simulink model "Damping_model"  (R2020a)
settings: Solver=VariableStepAuto  StartTime=0.0  StopTime=5  RelTol=1e-3  AbsTol=1e-3
undefined symbols (not defined in the file): b, b1, b2, b3, k, m
libraries: fl_lib x6, nesl_utility x3
settings Model: Creator=vltn0  LastModifiedBy=vltn0
settings SolverCC: AutoScaleAbsTol=off
settings DebuggingCC: SymbolicDimsDataTypeCodeGenerationDiagnostic=none
settings SFSimCC: CustomCodeUndefinedFunction=UseInterfaceOnly
settings SimscapeCC: SimscapeLogType=all  SimscapeLogSimulationStatistics=on  SimscapeLogDataHistory=10000

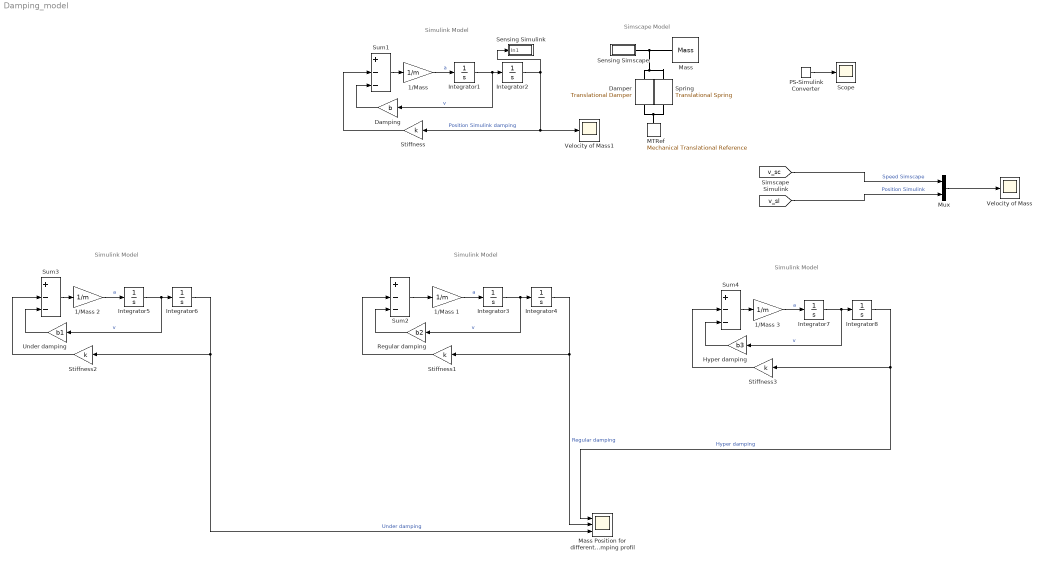
== system Damping_model ==
  note: Simulink Model
  note: Simscape Model
  note: Simulink Model
  note: Simulink Model
  note: Simulink Model
  1/Mass {,1..3} (4 alike) : Gain  Gain=1/m  SaturateOnIntegerOverflow=on  OutDataTypeStr=Inherit: Same as input  ParamDataTypeStr=Inherit: Same as input
  Damper : fl_lib/Mechanical/Translational Elements/Translational Damper  D=b N/(m/s)  v_specify=off  v_priority=High  v=0 m/s  v_nominal_specify=off  v_nominal_unit=m/s  v_nominal_value=1  f_specify=off  f_priority=High  f=0 N  f_nominal_specify=off  f_nominal_unit=N  f_nominal_value=1
  Damping : Gain  Gain=b  SaturateOnIntegerOverflow=on  OutDataTypeStr=Inherit: Same as input  ParamDataTypeStr=Inherit: Same as input
  Hyper damping : Gain  Gain=b3  SaturateOnIntegerOverflow=on  OutDataTypeStr=Inherit: Same as input  ParamDataTypeStr=Inherit: Same as input
  Integrator{1,3,5,7} (4 alike) : Integrator
  Integrator{2,4,6,8} (4 alike) : Integrator  InitialCondition=1
      settings: AttributesFormatString=x0 = %<InitialCondition> m
  MTRef : fl_lib/Mechanical/Translational Elements/Mechanical Translational Reference
  Mass : fl_lib/Mechanical/Translational Elements/Mass  mass=m kg  v_specify=off  v_priority=High  v=0 m/s  v_nominal_specify=off  v_nominal_unit=m/s  v_nominal_value=1  f_specify=off  f_priority=High  f=0 N  f_nominal_specify=off  f_nominal_unit=N  f_nominal_value=1
  Mass Position for different damping profil : Scope  NumInputPorts=3
  Mux : Mux  Inputs=3
  PS-Simulink Converter : nesl_utility/PS-Simulink Converter  PhysicalDomain=network_engine_domain  SubClassName=ps_output  LeftPortType=input  RightPortType=output  PseudoPeriodic=off  Frequencies=[]  Unit=inherit  AffineConversion=off
      settings: SourceProductBaseCode=MT,SS
  Regular damping : Gain  Gain=b2  SaturateOnIntegerOverflow=on  OutDataTypeStr=Inherit: Same as input  ParamDataTypeStr=Inherit: Same as input
  Scope : Scope
  Sensing Simscape : Subsystem
      mask Display: disp('v_sc')
  Sensing Simulink : Subsystem
      mask Display: disp('v_sl')
  Spring : fl_lib/Mechanical/Translational Elements/Translational Spring  spr_rate=k N/m  v_specify=off  v_priority=High  v=0 m/s  v_nominal_specify=off  v_nominal_unit=m/s  v_nominal_value=1  f_specify=off  f_priority=High  f=0 N  f_nominal_specify=off  f_nominal_unit=N  f_nominal_value=1  x_specify=on  x_priority=High  x=1 m  x_nominal_specify=off  x_nominal_unit=m  x_nominal_value=1
      settings: AttributesFormatString=x0 = %<x> %<x_unit>
  Stiffness{,1..3} (4 alike) : Gain  Gain=k  SaturateOnIntegerOverflow=on  OutDataTypeStr=Inherit: Same as input  ParamDataTypeStr=Inherit: Same as input
  Sum{1..4} (4 alike) : Sum  Inputs=+--  InputSameDT=on  SaturateOnIntegerOverflow=on  OutDataTypeStr=Inherit: Same as first input
  Under damping : Gain  Gain=b1  SaturateOnIntegerOverflow=on  OutDataTypeStr=Inherit: Same as input  ParamDataTypeStr=Inherit: Same as input
  Velocity of Mass : Scope
  Velocity of Mass1 : Scope
  wires:
  PS-Simulink Converter/1 -> Scope/1
  Integrator1/1 -> Integrator2/1, Damping/1  "v"
  Stiffness/1 -> Sum1/2
  Damping/1 -> Sum1/3
  Sum1/1 -> "1/Mass "/1
  "1/Mass "/1 -> Integrator1/1  "a"
  [v_sl] -> Mux/3  "Position Simulink"
  [v_sc] -> Mux/1  "Speed Simscape"
  Mux/1 -> Velocity of Mass/1
  Integrator2/1 -> Velocity of Mass1/1, Stiffness/1, Sensing Simulink/1(In1)  "Position Simulink damping"
  Sum2/1 -> 1/Mass 1/1
  Integrator4/1 -> Mass Position for different damping profil/2, Stiffness1/1  "Regular damping"
  Regular damping/1 -> Sum2/3
  Stiffness1/1 -> Sum2/2
  1/Mass 1/1 -> Integrator3/1  "a"
  Integrator3/1 -> Integrator4/1, Regular damping/1  "v"
  Sum3/1 -> 1/Mass 2/1
  Integrator6/1 -> Mass Position for different damping profil/3, Stiffness2/1  "Under damping"
  Under damping/1 -> Sum3/3
  Stiffness2/1 -> Sum3/2
  1/Mass 2/1 -> Integrator5/1  "a"
  Integrator5/1 -> Integrator6/1, Under damping/1  "v"
  Integrator7/1 -> Integrator8/1, Hyper damping/1  "v"
  1/Mass 3/1 -> Integrator7/1  "a"
  Sum4/1 -> 1/Mass 3/1
  Integrator8/1 -> Mass Position for different damping profil/1, Stiffness3/1  "Hyper damping"
  Stiffness3/1 -> Sum4/2
  Hyper damping/1 -> Sum4/3
  connections:
  Spring/RConn1 -- Damper/RConn1 -- MTRef/LConn1
  Spring/LConn1 -- Damper/LConn1 -- Sensing Simscape/LConn1 -- Mass/LConn1

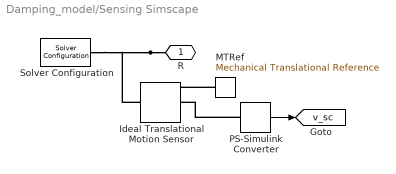
== system Damping_model/Sensing Simscape ==
  Ideal Translational Motion Sensor : fl_lib/Mechanical/Mechanical Sensors/Ideal Translational Motion Sensor  offset=1 m
  MTRef : fl_lib/Mechanical/Translational Elements/Mechanical Translational Reference
  PS-Simulink Converter : nesl_utility/PS-Simulink Converter  PhysicalDomain=network_engine_domain  SubClassName=ps_output  LeftPortType=input  RightPortType=output  PseudoPeriodic=off  Frequencies=[]  Unit=1  AffineConversion=off
  Solver Configuration : nesl_utility/Solver Configuration  PhysicalDomain=network_engine_domain  SubClassName=solver  LeftPortType=input  RightPortType=generic  Tones=[]  Harmonics=[]  SimulateNoise=off  Profile=off  UseLocalSampling=off  EnableSwitchedLinearOptims=on  FrequencyDomain=off  UseCCode=off  RelTol=0.001  AbsTol=1e-06  MinStep=1e-09  ToWorkspace=off  RevertToSquareIcSolve=off  NumHomotopyIterations=100  PhasorMode=off  PhasorModeNumHarmonics=1  DoDC=off  ResidualTolerance=1e-9  UseLocalSolver=off  LocalSolverChoice=NE_BACKWARD_EULER_ADVANCER  LocalSolverSampleTime=.001  DoFixedCost=off  MaxNonlinIter=12  MaxModeIter=2  LinearAlgebra=auto  EquationFormulation=NE_TIME_EF  DelaysMemoryBudget=1024  AutomaticFiltering=on  FilteringTimeConstant=0.001  PartitionStorageMethod=AS_NEEDED  PartitionMemoryBudget=1024  PartitionMethod=FAST
  R : PMIOPort  Side=Left
  tag scope: v_sc=global
  wires:
  PS-Simulink Converter/1 -> [v_sc]
  connections:
  MTRef/LConn1 -- Ideal Translational Motion Sensor/RConn1
  PS-Simulink Converter/LConn1 -- Ideal Translational Motion Sensor/RConn2
  R/RConn1 -- Ideal Translational Motion Sensor/LConn1 -- Solver Configuration/RConn1

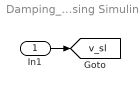
== system Damping_model/Sensing Simulink ==
  In1 : Inport
  tag scope: v_sl=global
  wires:
  In1/1 -> [v_sl]
